simulink model "saved3"  (R2018b)
settings: Solver=VariableStepAuto  StartTime=0.0  StopTime=10.0  RelTol=1e-3
libraries: simulink x95, powerlib x8, powerlib_meascontrol x2
(part 6 of 6)

== matlab function saved3/全观测角速度闭环控制/controller1/MATLAB Function1 ==
  data: u input; y output; t input
function y = fcn(u,t)
startTime=0.2;
if t>startTime
    y=u;
else
    y=0;
end

== matlab function saved3/离散化半成品/PSMS/PMSM dq/MATLAB Function1 ==
  data: i1 input; dw output; i2 input; w input; torE input
function dw = fcn(i1,i2,w,torE)
L1=1e-3; L2=1.4e-3;
phi=0.05;
J=1e-3;
xi=5e-4;

dw = 1/J*(1.5*(phi*i2+(L1-L2)*i1*i2)-xi*w-torE);

== matlab function saved3/全观测角速度闭环控制/w estimater1/MATLAB Function ==
  data: Ea input; y output; Eb input
function y = fcn(Ea,Eb)
if Ea^2+Eb^2<1e-1
    y=0;
else
    y = atan2(Ea,-Eb);
end

== matlab function saved3/全观测角速度闭环控制/w estimater1/clack ==
  data: ia input; iap output; ib input; ic input; ibe output
function [iap,ibe] = fcn(ia,ib,ic)
clack=2/3*[1 -1/2 -1/2;0 sqrt(3)/2 -sqrt(3)/2];
temp=clack*[ia;ib;ic];
iap=temp(1);
ibe=temp(2);

== matlab function saved3/全观测角速度闭环控制/w estimater1/invpark ==
  data: u1 input; ua output; u2 input; ub output; t input
function [ua,ub] = fcn(u1,u2,t)
invPark=[cos(t) -sin(t);sin(t) cos(t)];
temp=invPark*[u1;u2];
ua=temp(1);
ub=temp(2);

== matlab function saved3/离散化半成品/PSMS/clack & park ==
  data: ua input; u1 output; ub input; uc input; t input; u2 output
function [u1,u2] = fcn(ua,ub,uc,t)
clack=2/3*[1 -1/2 -1/2;0 sqrt(3)/2 -sqrt(3)/2];
park=[cos(t) sin(t);-sin(t) cos(t)];
temp=park*clack*[ua;ub;uc];
u1=temp(1);
u2=temp(2);

== matlab function saved3/离散化半成品/PSMS/inv(clack & park) ==
  data: u1 input; ua output; u2 input; t input; ub output; uc output
function [ua,ub,uc] = fcn(u1,u2,t)
invClack=3/2*[2/3 0;-1/3 sqrt(3)/3;-1/3 -sqrt(3)/3];
invPark=[cos(t) -sin(t);sin(t) cos(t)];
temp=invClack*invPark*[u1;u2];
ua=temp(1);
ub=temp(2);
uc=temp(3);

== matlab function saved3/离散化半成品/clack & park2 ==
  data: ua input; u1 output; ub input; uc input; t input; u2 output
function [u1,u2] = fcn(ua,ub,uc,t)
clack=2/3*[1 -1/2 -1/2;0 sqrt(3)/2 -sqrt(3)/2];
park=[cos(t) sin(t);-sin(t) cos(t)];
temp=park*clack*[ua;ub;uc];
u1=temp(1);
u2=temp(2);

== matlab function saved3/离散化半成品/controller/MATLAB Function ==
  data: wloop input; Vdirect input; Switch input; t input; out output
function out = fcn(wloop,Vdirect,Switch,t)
step1time=0.1;
step2time=0.2;
Ustart=1;
direction=1;
if t<step1time
    y=0;
else
    switch Switch
        case 0
            if t<step2time
                y=Ustart*direction;
            else
                y=wloop;
            end
        case 1
            y=Vdirect;
        otherwise
            y=0;
    end
end
out=y;

== matlab function saved3/离散化半成品/controller/MATLAB Function1 ==
  data: u input; y output; t input
function y = fcn(u,t)
startTime=0.2;
if t>startTime
    y=u;
else
    y=0;
end

== matlab function saved3/离散化半成品/inject estimater(digital)/鉴幅鉴相器(可选快速门滑窗) ==
  data: S1 input; A1 output; A2 output; S2 input; DP output; Fre input
function [A1,A2, DP] = fcn(S1,S2,Fre)
Ts=1e-4; %采样时间，其倒数需大于10倍探测信号频率
detPsi=Fre; %探测频率.需采样完整周期整数倍
LowPsi=Fre; %输入信号中的最低显著频率，若探测频率远大于该项，需前置高通滤波器
bufsize=2/LowPsi/Ts;
winSize=1; %滑窗步长
complexStyle=1+1j;
persistent buf1 buf2 round outBuf corebuf gate
if isempty(buf1)||isempty(round)
    buf1=zeros(1,bufsize);
    buf2=zeros(1,bufsize);
    corebuf=zeros(1,bufsize,'like',complexStyle);
    round=0;
    outBuf=[0,0,0];
    gate=0;
end
% 数据读取
if round>=bufsize
    round=0;
    gate=1;
end
buf1(round+1)=S1;
buf2(round+1)=S2;
% 数据处理
corebuf(round+1)=exp(-2*pi*1j*detPsi*round*Ts)*Ts;
if gate==1
    if mod(round+1,winSize)==0
        F1=0+0j;F2=0+0j;
        for n=0:bufsize-1
            F1=F1+buf1(n+1)*corebuf(n+1);
            F2=F2+buf2(n+1)*corebuf(n+1);
        end
        F1=F1*2/bufsize/Ts;F2=F2*2/bufsize/Ts;
        outBuf(1)=norm(F1);outBuf(2)=norm(F2);
        outBuf(3)=angle(F2/F1)*180/pi; %S2超前S1的相位
    end
end
% 更新与输出
round=round+1;
A1=outBuf(1);A2=outBuf(2);
DP=outBuf(3);

== matlab function saved3/离散化半成品/inject estimater(digital)/锁相器 ==
  data: u input; the output; w output
function [the,w] = fcn(u)
% PI控制器部分
ts=1e-4;
kp=4; ki=350;
persistent intg
if isempty(intg)
    intg=0;
end
intg=intg+u*ts;
w = kp*u+ki*intg;

% 积分器部分
persistent intg2
if isempty(intg2)
    intg2=0;
end
intg2=intg2+w*ts;
the = intg2;

== matlab function saved3/离散化半成品/inv(clack & park)1 ==
  data: u1 input; ua output; u2 input; t input; ub output; uc output
function [ua,ub,uc] = fcn(u1,u2,t)
invClack=3/2*[2/3 0;-1/3 sqrt(3)/3;-1/3 -sqrt(3)/3];
invPark=[cos(t) -sin(t);sin(t) cos(t)];
temp=invClack*invPark*[u1;u2];
ua=temp(1);
ub=temp(2);
uc=temp(3);

== matlab function saved3/离散化半成品/w estimater/MATLAB Function ==
  data: Ea input; y output; Eb input
function y = fcn(Ea,Eb)
if Ea^2+Eb^2<1e-1
    y=0;
else
    y = atan2(Ea,-Eb);
end

== matlab function saved3/离散化半成品/w estimater/clack ==
  data: ia input; iap output; ib input; ic input; ibe output
function [iap,ibe] = fcn(ia,ib,ic)
clack=2/3*[1 -1/2 -1/2;0 sqrt(3)/2 -sqrt(3)/2];
temp=clack*[ia;ib;ic];
iap=temp(1);
ibe=temp(2);

== matlab function saved3/离散化半成品/w estimater/invpark ==
  data: u1 input; ua output; u2 input; ub output; t input
function [ua,ub] = fcn(u1,u2,t)
invPark=[cos(t) -sin(t);sin(t) cos(t)];
temp=invPark*[u1;u2];
ua=temp(1);
ub=temp(2);

== matlab function saved3/离散化半成品/电流采样/A//D转换 10KHz2 ==
  data: u input; y output
function y = fcn(u)
bina=16; %二进制位数
deci=2; %小数位数
Max=2^bina;
uper=Max/10^deci/2;
out=fix(u*10^deci+0.5)/10^deci;
y = min(uper,abs(out))*sign(out);

== matlab function saved3/离散化半成品/电流采样/A//D转换 10KHz3 ==
  data: u input; y output
function y = fcn(u)
bina=16; %二进制位数
deci=2; %小数位数
Max=2^bina;
uper=Max/10^deci/2;
out=fix(u*10^deci+0.5)/10^deci;
y = min(uper,abs(out))*sign(out);

== matlab function saved3/离散化半成品/电流采样/A//D转换 10KHz4 ==
  data: u input; y output
function y = fcn(u)
bina=16; %二进制位数
deci=2; %小数位数
Max=2^bina;
uper=Max/10^deci/2;
out=fix(u*10^deci+0.5)/10^deci;
y = min(uper,abs(out))*sign(out);

== matlab function saved3/离散化半成品/电流采样/一阶滤波器40kHz1 ==
  data: u input; y output
function y = fcn(u)
ts=2.5e-5;
N=16000; %截止角频率
persistent xK_1
if isempty(xK_1)
    xK_1=0;
end
x=ts*N*(u-xK_1)+xK_1;
xK_1=x;
y = x;

== matlab function saved3/离散化半成品/电流采样/一阶滤波器40kHz2 ==
  data: u input; y output
function y = fcn(u)
ts=2.5e-5;
N=16000; %截止角频率
persistent xK_1
if isempty(xK_1)
    xK_1=0;
end
x=ts*N*(u-xK_1)+xK_1;
xK_1=x;
y = x;

== matlab function saved3/离散化半成品/电流采样/一阶滤波器40kHz3 ==
  data: u input; y output
function y = fcn(u)
ts=2.5e-5;
N=16000; %截止角频率
persistent xK_1
if isempty(xK_1)
    xK_1=0;
end
x=ts*N*(u-xK_1)+xK_1;
xK_1=x;
y = x;

== matlab function saved3/离散化半成品/2pi 限制2 ==
  data: u input; y output
function y = fcn(u)

y = mod((u+pi),2*pi)-pi;

== matlab function saved3/离散化半成品/MATLAB Function1 ==
  data: hfi input; mlo input; theHat output; t input
function theHat = fcn(hfi, mlo, t)
if t>0.4
    theHat=mlo;
else
    theHat=hfi;
end

== matlab function saved3/离散化半成品/MATLAB Function4 ==
  data: t input; y output
function y = fcn(t)
t=t-0.05;
y = 0*(t<=0.05)+500*(t-0.05)*(0.05<t&&t<=0.35)+(250*(t-0.35)+150)*(0.35<t&&t<=0.55)+200*(t>0.55);

== matlab function saved3/离散化半成品/PSMS1/PMSM dq/MATLAB Function ==
  data: u1 input; di1 output; u2 input; i1 input; i2 input; w input; di2 output
function [di1,di2] = fcn(u1,u2,i1,i2,w)
R=0.1; L1=1e-3; L2=1.4e-3;
phi=0.05;

A=[R/L1 -L2/L1*w;L1/L2*w R/L2];
Y=[1/L1 0;0 1/L2];
I=[i1;i2];
U=[u1;u2];

dI=-A*I+Y*U-phi*w*[0;1/L2];
di1=dI(1);
di2=dI(2);

== matlab function saved3/离散化半成品/PSMS1/PMSM dq/MATLAB Function1 ==
  data: i1 input; dw output; i2 input; w input; torE input
function dw = fcn(i1,i2,w,torE)
L1=1e-3; L2=1.4e-3;
phi=0.05;
J=1e-3;
xi=5e-4;

dw = 1/J*(1.5*(phi*i2+(L1-L2)*i1*i2)-xi*w-torE);

== matlab function saved3/离散化半成品/PSMS1/clack & park ==
  data: ua input; u1 output; ub input; uc input; t input; u2 output
function [u1,u2] = fcn(ua,ub,uc,t)
clack=2/3*[1 -1/2 -1/2;0 sqrt(3)/2 -sqrt(3)/2];
park=[cos(t) sin(t);-sin(t) cos(t)];
temp=park*clack*[ua;ub;uc];
u1=temp(1);
u2=temp(2);

== matlab function saved3/离散化半成品/PSMS1/inv(clack & park) ==
  data: u1 input; ua output; u2 input; t input; ub output; uc output
function [ua,ub,uc] = fcn(u1,u2,t)
invClack=3/2*[2/3 0;-1/3 sqrt(3)/3;-1/3 -sqrt(3)/3];
invPark=[cos(t) -sin(t);sin(t) cos(t)];
temp=invClack*invPark*[u1;u2];
ua=temp(1);
ub=temp(2);
uc=temp(3);

== matlab function saved3/离散化半成品/controller1/MATLAB Function ==
  data: wloop input; Vdirect input; Switch input; t input; out output
function out = fcn(wloop,Vdirect,Switch,t)
step1time=0.1;
step2time=0.2;
Ustart=1;
direction=1;
if t<step1time
    y=0;
else
    switch Switch
        case 0
            if t<step2time
                y=Ustart*direction;
            else
                y=wloop;
            end
        case 1
            y=Vdirect;
        otherwise
            y=0;
    end
end
out=y;

== matlab function saved3/离散化半成品/controller1/MATLAB Function1 ==
  data: u input; y output; t input
function y = fcn(u,t)
startTime=0.2;
if t>startTime
    y=u;
else
    y=0;
end

== matlab function saved3/离散化半成品/controller1/MATLAB Function2 ==
  data: gate input; u input; y output
function y = fcn(gate,u)
if gate<100
    y=u;
else
    y=0;
end

== matlab function saved3/离散化半成品/controller1/clack & park1 ==
  data: ua input; u1 output; ub input; uc input; t input; u2 output
function [u1,u2] = fcn(ua,ub,uc,t)
clack=2/3*[1 -1/2 -1/2;0 sqrt(3)/2 -sqrt(3)/2];
park=[cos(t) sin(t);-sin(t) cos(t)];
temp=park*clack*[ua;ub;uc];
u1=temp(1);
u2=temp(2);

== matlab function saved3/离散化半成品/current seperator/电流采样/A//D转换 10KHz2 ==
  data: u input; y output
function y = fcn(u)
bina=16; %二进制位数
deci=3; %小数位数
Max=2^bina;
uper=Max/10^deci/2;
out=fix(u*10^deci+0.5)/10^deci;
y = min(uper,abs(out))*sign(out);

== matlab function saved3/离散化半成品/current seperator/电流采样/A//D转换 10KHz3 ==
  data: u input; y output
function y = fcn(u)
bina=16; %二进制位数
deci=3; %小数位数
Max=2^bina;
uper=Max/10^deci/2;
out=fix(u*10^deci+0.5)/10^deci;
y = min(uper,abs(out))*sign(out);

== matlab function saved3/离散化半成品/current seperator/电流采样/A//D转换 10KHz4 ==
  data: u input; y output
function y = fcn(u)
bina=16; %二进制位数
deci=3; %小数位数
Max=2^bina;
uper=Max/10^deci/2;
out=fix(u*10^deci+0.5)/10^deci;
y = min(uper,abs(out))*sign(out);

== matlab function saved3/离散化半成品/current seperator/电流采样1/A//D转换 10KHz2 ==
  data: u input; y output
function y = fcn(u)
bina=16; %二进制位数
deci=2; %小数位数
Max=2^bina;
uper=Max/10^deci/2;
out=fix(u*10^deci+0.5)/10^deci;
y = min(uper,abs(out))*sign(out);

== matlab function saved3/离散化半成品/current seperator/电流采样1/A//D转换 10KHz3 ==
  data: u input; y output
function y = fcn(u)
bina=16; %二进制位数
deci=2; %小数位数
Max=2^bina;
uper=Max/10^deci/2;
out=fix(u*10^deci+0.5)/10^deci;
y = min(uper,abs(out))*sign(out);

== matlab function saved3/离散化半成品/current seperator/电流采样1/A//D转换 10KHz4 ==
  data: u input; y output
function y = fcn(u)
bina=16; %二进制位数
deci=2; %小数位数
Max=2^bina;
uper=Max/10^deci/2;
out=fix(u*10^deci+0.5)/10^deci;
y = min(uper,abs(out))*sign(out);

== matlab function saved3/离散化半成品/inject estimater(digital)1/clack & park2 ==
  data: ua input; u1 output; ub input; uc input; t input; u2 output
function [u1,u2] = fcn(ua,ub,uc,t)
clack=2/3*[1 -1/2 -1/2;0 sqrt(3)/2 -sqrt(3)/2];
park=[cos(t) sin(t);-sin(t) cos(t)];
temp=park*clack*[ua;ub;uc];
u1=temp(1);
u2=temp(2);

== matlab function saved3/离散化半成品/inject estimater(digital)1/鉴幅鉴相器(可选快速门滑窗)1 ==
  data: S1 input; A1 output; A2 output; S2 input; DP output; Fre input
function [A1,A2, DP] = fcn(S1,S2,Fre)
Ts=1e-4; %采样时间，其倒数需大于10倍探测信号频率
detPsi=Fre; %探测频率.需采样完整周期整数倍
LowPsi=Fre; %输入信号中的最低显著频率，若探测频率远大于该项，需前置高通滤波器
bufsize=2/LowPsi/Ts;
winSize=1; %滑窗步长
complexStyle=1+1j;
persistent buf1 buf2 round outBuf corebuf gate
if isempty(buf1)||isempty(round)
    buf1=zeros(1,bufsize);
    buf2=zeros(1,bufsize);
    corebuf=zeros(1,bufsize,'like',complexStyle);
    round=0;
    outBuf=[0,0,0];
    gate=0;
end
% 数据读取
if round>=bufsize
    round=0;
    gate=1;
end
buf1(round+1)=S1;
buf2(round+1)=S2;
% 数据处理
corebuf(round+1)=exp(-2*pi*1j*detPsi*round*Ts)*Ts;
if gate==1
    if mod(round+1,winSize)==0
        F1=0+0j;F2=0+0j;
        for n=0:bufsize-1
            F1=F1+buf1(n+1)*corebuf(n+1);
            F2=F2+buf2(n+1)*corebuf(n+1);
        end
        F1=F1*2/bufsize/Ts;F2=F2*2/bufsize/Ts;
        outBuf(1)=norm(F1);outBuf(2)=norm(F2);
        outBuf(3)=angle(F2/F1)*180/pi; %S2超前S1的相位
    end
end
% 更新与输出
round=round+1;
A1=outBuf(1);A2=outBuf(2);
DP=outBuf(3);

== matlab function saved3/离散化半成品/inject estimater(digital)1/锁相器1 ==
  data: u input; the output; w output
function [the,w] = fcn(u)
% PI控制器部分
ts=1e-4;
kp=4; ki=350;
persistent intg
if isempty(intg)
    intg=0;
end
intg=intg+u*ts;
w = kp*u+ki*intg;

% 积分器部分
persistent intg2
if isempty(intg2)
    intg2=0;
end
intg2=intg2+w*ts;
the = intg2;

== matlab function saved3/离散化半成品/inv(clack & park)2 ==
  data: u1 input; ua output; u2 input; t input; ub output; uc output
function [ua,ub,uc] = fcn(u1,u2,t)
invClack=3/2*[2/3 0;-1/3 sqrt(3)/3;-1/3 -sqrt(3)/3];
invPark=[cos(t) -sin(t);sin(t) cos(t)];
temp=invClack*invPark*[u1;u2];
ua=temp(1);
ub=temp(2);
uc=temp(3);

== matlab function saved3/离散化半成品/w estimater1/clack1 ==
  data: ia input; iap output; ib input; ic input; ibe output
function [iap,ibe] = fcn(ia,ib,ic)
clack=2/3*[1 -1/2 -1/2;0 sqrt(3)/2 -sqrt(3)/2];
temp=clack*[ia;ib;ic];
iap=temp(1);
ibe=temp(2);

== matlab function saved3/离散化半成品/2pi 限制3 ==
  data: u input; y output
function y = fcn(u)

y = mod((u+pi),2*pi)-pi;

== matlab function saved3/离散化半成品/MATLAB Function2 ==
  data: t input; y output
function y = fcn(t)
t=t-0.05;
y = 0*(t<=0.05)+500*(t-0.05)*(0.05<t&&t<=0.35)+(250*(t-0.35)+150)*(0.35<t&&t<=0.55)+200*(t>0.55);

== matlab function saved3/离散化半成品/PSMS2/PMSM dq/MATLAB Function ==
  data: u1 input; di1 output; u2 input; i1 input; i2 input; w input; di2 output
function [di1,di2] = fcn(u1,u2,i1,i2,w)
R=0.1; L1=1e-3; L2=1.4e-3;
phi=0.05;

A=[R/L1 -L2/L1*w;L1/L2*w R/L2];
Y=[1/L1 0;0 1/L2];
I=[i1;i2];
U=[u1;u2];

dI=-A*I+Y*U-phi*w*[0;1/L2];
di1=dI(1);
di2=dI(2);

== matlab function saved3/离散化半成品/PSMS2/PMSM dq/MATLAB Function1 ==
  data: i1 input; dw output; i2 input; w input; torE input
function dw = fcn(i1,i2,w,torE)
L1=1e-3; L2=1.4e-3;
phi=0.05;
J=1e-3;
xi=5e-4;

dw = 1/J*(1.5*(phi*i2+(L1-L2)*i1*i2)-xi*w-torE);

== matlab function saved3/离散化半成品/PSMS2/clack & park ==
  data: ua input; u1 output; ub input; uc input; t input; u2 output
function [u1,u2] = fcn(ua,ub,uc,t)
clack=2/3*[1 -1/2 -1/2;0 sqrt(3)/2 -sqrt(3)/2];
park=[cos(t) sin(t);-sin(t) cos(t)];
temp=park*clack*[ua;ub;uc];
u1=temp(1);
u2=temp(2);

== matlab function saved3/离散化半成品/PSMS2/inv(clack & park) ==
  data: u1 input; ua output; u2 input; t input; ub output; uc output
function [ua,ub,uc] = fcn(u1,u2,t)
invClack=3/2*[2/3 0;-1/3 sqrt(3)/3;-1/3 -sqrt(3)/3];
invPark=[cos(t) -sin(t);sin(t) cos(t)];
temp=invClack*invPark*[u1;u2];
ua=temp(1);
ub=temp(2);
uc=temp(3);

== matlab function saved3/离散化半成品/Subsystem/电流采样/A//D转换 10KHz2 ==
  data: u input; y output
function y = fcn(u)
bina=16; %二进制位数
deci=2; %小数位数
Max=2^bina;
uper=Max/10^deci/2;
out=fix(u*10^deci+0.5)/10^deci;
y = min(uper,abs(out))*sign(out);

== matlab function saved3/离散化半成品/Subsystem/电流采样/A//D转换 10KHz3 ==
  data: u input; y output
function y = fcn(u)
bina=16; %二进制位数
deci=2; %小数位数
Max=2^bina;
uper=Max/10^deci/2;
out=fix(u*10^deci+0.5)/10^deci;
y = min(uper,abs(out))*sign(out);

== matlab function saved3/离散化半成品/Subsystem/电流采样/A//D转换 10KHz4 ==
  data: u input; y output
function y = fcn(u)
bina=16; %二进制位数
deci=2; %小数位数
Max=2^bina;
uper=Max/10^deci/2;
out=fix(u*10^deci+0.5)/10^deci;
y = min(uper,abs(out))*sign(out);

== matlab function saved3/离散化半成品/Subsystem/电流采样/一阶滤波器40kHz1 ==
  data: u input; y output
function y = fcn(u)
ts=2.5e-5;
N=16000; %截止角频率
persistent xK_1
if isempty(xK_1)
    xK_1=0;
end
x=ts*N*(u-xK_1)+xK_1;
xK_1=x;
y = x;

== matlab function saved3/离散化半成品/Subsystem/电流采样/一阶滤波器40kHz2 ==
  data: u input; y output
function y = fcn(u)
ts=2.5e-5;
N=16000; %截止角频率
persistent xK_1
if isempty(xK_1)
    xK_1=0;
end
x=ts*N*(u-xK_1)+xK_1;
xK_1=x;
y = x;

== matlab function saved3/离散化半成品/Subsystem/电流采样/一阶滤波器40kHz3 ==
  data: u input; y output
function y = fcn(u)
ts=2.5e-5;
N=16000; %截止角频率
persistent xK_1
if isempty(xK_1)
    xK_1=0;
end
x=ts*N*(u-xK_1)+xK_1;
xK_1=x;
y = x;

== matlab function saved3/离散化半成品/clack & park1 ==
  data: ua input; u1 output; ub input; uc input; t input; u2 output
function [u1,u2] = fcn(ua,ub,uc,t)
clack=2/3*[1 -1/2 -1/2;0 sqrt(3)/2 -sqrt(3)/2];
park=[cos(t) sin(t);-sin(t) cos(t)];
temp=park*clack*[ua;ub;uc];
u1=temp(1);
u2=temp(2);

== matlab function saved3/离散化半成品/controller2/MATLAB Function ==
  data: wloop input; Vdirect input; Switch input; t input; out output
function out = fcn(wloop,Vdirect,Switch,t)
step1time=0.1;
step2time=0.2;
Ustart=1;
direction=1;
if t<step1time
    y=0;
else
    switch Switch
        case 0
            if t<step2time
                y=Ustart*direction;
            else
                y=wloop;
            end
        case 1
            y=Vdirect;
        otherwise
            y=0;
    end
end
out=y;

== matlab function saved3/离散化半成品/controller2/MATLAB Function1 ==
  data: u input; y output; t input
function y = fcn(u,t)
startTime=0.2;
if t>startTime
    y=u;
else
    y=0;
end

== matlab function saved3/离散化半成品/inject estimater(digital)2/clack & park2 ==
  data: ua input; u1 output; ub input; uc input; t input; u2 output
function [u1,u2] = fcn(ua,ub,uc,t)
clack=2/3*[1 -1/2 -1/2;0 sqrt(3)/2 -sqrt(3)/2];
park=[cos(t) sin(t);-sin(t) cos(t)];
temp=park*clack*[ua;ub;uc];
u1=temp(1);
u2=temp(2);

== matlab function saved3/离散化半成品/inject estimater(digital)2/鉴幅鉴相器(可选快速门滑窗)1 ==
  data: S1 input; A1 output; A2 output; S2 input; DP output; Fre input
function [A1,A2, DP] = fcn(S1,S2,Fre)
Ts=1e-4; %采样时间，其倒数需大于10倍探测信号频率
detPsi=Fre; %探测频率.需采样完整周期整数倍
LowPsi=Fre; %输入信号中的最低显著频率，若探测频率远大于该项，需前置高通滤波器
bufsize=2/LowPsi/Ts;
winSize=1; %滑窗步长
complexStyle=1+1j;
persistent buf1 buf2 round outBuf corebuf gate
if isempty(buf1)||isempty(round)
    buf1=zeros(1,bufsize);
    buf2=zeros(1,bufsize);
    corebuf=zeros(1,bufsize,'like',complexStyle);
    round=0;
    outBuf=[0,0,0];
    gate=0;
end
% 数据读取
if round>=bufsize
    round=0;
    gate=1;
end
buf1(round+1)=S1;
buf2(round+1)=S2;
% 数据处理
corebuf(round+1)=exp(-2*pi*1j*detPsi*round*Ts)*Ts;
if gate==1
    if mod(round+1,winSize)==0
        F1=0+0j;F2=0+0j;
        for n=0:bufsize-1
            F1=F1+buf1(n+1)*corebuf(n+1);
            F2=F2+buf2(n+1)*corebuf(n+1);
        end
        F1=F1*2/bufsize/Ts;F2=F2*2/bufsize/Ts;
        outBuf(1)=norm(F1);outBuf(2)=norm(F2);
        outBuf(3)=angle(F2/F1)*180/pi; %S2超前S1的相位
    end
end
% 更新与输出
round=round+1;
A1=outBuf(1);A2=outBuf(2);
DP=outBuf(3);

== matlab function saved3/离散化半成品/inject estimater(digital)2/锁相器1 ==
  data: u input; the output; w output
function [the,w] = fcn(u)
% PI控制器部分
ts=1e-4;
kp=4; ki=350;
persistent intg
if isempty(intg)
    intg=0;
end
intg=intg+u*ts;
w = kp*u+ki*intg;

% 积分器部分
persistent intg2
if isempty(intg2)
    intg2=0;
end
intg2=intg2+w*ts;
the = intg2;

== matlab function saved3/离散化半成品/inv(clack & park)3 ==
  data: u1 input; ua output; u2 input; t input; ub output; uc output
function [ua,ub,uc] = fcn(u1,u2,t)
invClack=3/2*[2/3 0;-1/3 sqrt(3)/3;-1/3 -sqrt(3)/3];
invPark=[cos(t) -sin(t);sin(t) cos(t)];
temp=invClack*invPark*[u1;u2];
ua=temp(1);
ub=temp(2);
uc=temp(3);

== matlab function saved3/离散化半成品/w estimater2/MATLAB Function ==
  data: Ea input; y output; Eb input
function y = fcn(Ea,Eb)
if Ea^2+Eb^2<1e-1
    y=0;
else
    y = atan2(Ea,-Eb);
end

== matlab function saved3/离散化半成品/w estimater2/clack ==
  data: ia input; iap output; ib input; ic input; ibe output
function [iap,ibe] = fcn(ia,ib,ic)
clack=2/3*[1 -1/2 -1/2;0 sqrt(3)/2 -sqrt(3)/2];
temp=clack*[ia;ib;ic];
iap=temp(1);
ibe=temp(2);

== matlab function saved3/离散化半成品/w estimater2/invpark ==
  data: u1 input; ua output; u2 input; ub output; t input
function [ua,ub] = fcn(u1,u2,t)
invPark=[cos(t) -sin(t);sin(t) cos(t)];
temp=invPark*[u1;u2];
ua=temp(1);
ub=temp(2);

== matlab function saved3/离散化半成品/电流采样1/A//D转换 10KHz2 ==
  data: u input; y output
function y = fcn(u)
bina=16; %二进制位数
deci=2; %小数位数
Max=2^bina;
uper=Max/10^deci/2;
out=fix(u*10^deci+0.5)/10^deci;
y = min(uper,abs(out))*sign(out);

== matlab function saved3/离散化半成品/电流采样1/A//D转换 10KHz3 ==
  data: u input; y output
function y = fcn(u)
bina=16; %二进制位数
deci=2; %小数位数
Max=2^bina;
uper=Max/10^deci/2;
out=fix(u*10^deci+0.5)/10^deci;
y = min(uper,abs(out))*sign(out);

== matlab function saved3/离散化半成品/电流采样1/A//D转换 10KHz4 ==
  data: u input; y output
function y = fcn(u)
bina=16; %二进制位数
deci=2; %小数位数
Max=2^bina;
uper=Max/10^deci/2;
out=fix(u*10^deci+0.5)/10^deci;
y = min(uper,abs(out))*sign(out);

== matlab function saved3/离散化半成品/电流采样1/一阶滤波器40kHz1 ==
  data: u input; y output
function y = fcn(u)
ts=2.5e-5;
N=16000; %截止角频率
persistent xK_1
if isempty(xK_1)
    xK_1=0;
end
x=ts*N*(u-xK_1)+xK_1;
xK_1=x;
y = x;

== matlab function saved3/全观测角速度闭环控制/controller/MATLAB Function1 ==
  data: u input; y output; t input
function y = fcn(u,t)
startTime=0.2;
if t>startTime
    y=u;
else
    y=0;
end

== matlab function saved3/离散化半成品/电流采样1/一阶滤波器40kHz2 ==
  data: u input; y output
function y = fcn(u)
ts=2.5e-5;
N=16000; %截止角频率
persistent xK_1
if isempty(xK_1)
    xK_1=0;
end
x=ts*N*(u-xK_1)+xK_1;
xK_1=x;
y = x;

== matlab function saved3/离散化半成品/电流采样1/一阶滤波器40kHz3 ==
  data: u input; y output
function y = fcn(u)
ts=2.5e-5;
N=16000; %截止角频率
persistent xK_1
if isempty(xK_1)
    xK_1=0;
end
x=ts*N*(u-xK_1)+xK_1;
xK_1=x;
y = x;

== matlab function saved3/离散化半成品/MATLAB Function ==
  data: Inj input; theHat output; Emf input; wHat input; t input
function theHat = fcn(Inj,Emf, wHat,t)

if t>0.4
    theHat=Emf;
else
    theHat=Inj;
end

== matlab function saved3/离散化半成品/MATLAB Function3 ==
  data: t input; y output
function y = fcn(t)
t=t-0.05;
y = 0*(t<=0.05)+500*(t-0.05)*(0.05<t&&t<=0.35)+(250*(t-0.35)+150)*(0.35<t&&t<=0.55)+200*(t>0.55);

== matlab function saved3/全观测角速度闭环控制/PSMS/PMSM dq/MATLAB Function ==
  data: u1 input; di1 output; u2 input; i1 input; i2 input; w input; di2 output
function [di1,di2] = fcn(u1,u2,i1,i2,w)
R=0.1; L1=1e-3; L2=1.4e-3;
phi=0.05;

A=[R/L1 -L2/L1*w;L1/L2*w R/L2];
Y=[1/L1 0;0 1/L2];
I=[i1;i2];
U=[u1;u2];

dI=-A*I+Y*U-phi*w*[0;1/L2];
di1=dI(1);
di2=dI(2);

== matlab function saved3/全观测角速度闭环控制/PSMS/PMSM dq/MATLAB Function1 ==
  data: i1 input; dw output; i2 input; w input; torE input
function dw = fcn(i1,i2,w,torE)
L1=1e-3; L2=1.4e-3;
phi=0.05;
J=1e-3;
xi=5e-4;

dw = 1/J*(1.5*(phi*i2+(L1-L2)*i1*i2)-xi*w-torE);

== matlab function saved3/全观测角速度闭环控制/PSMS/clack & park ==
  data: ua input; u1 output; ub input; uc input; t input; u2 output
function [u1,u2] = fcn(ua,ub,uc,t)
clack=2/3*[1 -1/2 -1/2;0 sqrt(3)/2 -sqrt(3)/2];
park=[cos(t) sin(t);-sin(t) cos(t)];
temp=park*clack*[ua;ub;uc];
u1=temp(1);
u2=temp(2);

== matlab function saved3/全观测角速度闭环控制/PSMS/inv(clack & park) ==
  data: u1 input; ua output; u2 input; t input; ub output; uc output
function [ua,ub,uc] = fcn(u1,u2,t)
invClack=3/2*[2/3 0;-1/3 sqrt(3)/3;-1/3 -sqrt(3)/3];
invPark=[cos(t) -sin(t);sin(t) cos(t)];
temp=invClack*invPark*[u1;u2];
ua=temp(1);
ub=temp(2);
uc=temp(3);

== matlab function saved3/全观测角速度闭环控制/clack & park2 ==
  data: ua input; u1 output; ub input; uc input; t input; u2 output
function [u1,u2] = fcn(ua,ub,uc,t)
clack=2/3*[1 -1/2 -1/2;0 sqrt(3)/2 -sqrt(3)/2];
park=[cos(t) sin(t);-sin(t) cos(t)];
temp=park*clack*[ua;ub;uc];
u1=temp(1);
u2=temp(2);

== matlab function saved3/离散化半成品/PSMS3/PMSM dq/MATLAB Function ==
  data: u1 input; di1 output; u2 input; i1 input; i2 input; w input; di2 output
function [di1,di2] = fcn(u1,u2,i1,i2,w)
R=0.1; L1=1e-3; L2=1.4e-3;
phi=0.05;

A=[R/L1 -L2/L1*w;L1/L2*w R/L2];
Y=[1/L1 0;0 1/L2];
I=[i1;i2];
U=[u1;u2];

dI=-A*I+Y*U-phi*w*[0;1/L2];
di1=dI(1);
di2=dI(2);

== matlab function saved3/全观测角速度闭环控制/inv(clack & park)1 ==
  data: u1 input; ua output; u2 input; t input; ub output; uc output
function [ua,ub,uc] = fcn(u1,u2,t)
invClack=3/2*[2/3 0;-1/3 sqrt(3)/3;-1/3 -sqrt(3)/3];
invPark=[cos(t) -sin(t);sin(t) cos(t)];
temp=invClack*invPark*[u1;u2];
ua=temp(1);
ub=temp(2);
uc=temp(3);

== matlab function saved3/离散化半成品/PSMS3/PMSM dq/MATLAB Function1 ==
  data: i1 input; dw output; i2 input; w input; torE input
function dw = fcn(i1,i2,w,torE)
L1=1e-3; L2=1.4e-3;
phi=0.05;
J=1e-3;
xi=5e-4;

dw = 1/J*(1.5*(phi*i2+(L1-L2)*i1*i2)-xi*w-torE);

== matlab function saved3/离散化半成品/PSMS3/clack & park ==
  data: ua input; u1 output; ub input; uc input; t input; u2 output
function [u1,u2] = fcn(ua,ub,uc,t)
clack=2/3*[1 -1/2 -1/2;0 sqrt(3)/2 -sqrt(3)/2];
park=[cos(t) sin(t);-sin(t) cos(t)];
temp=park*clack*[ua;ub;uc];
u1=temp(1);
u2=temp(2);

== matlab function saved3/离散化半成品/PSMS3/inv(clack & park) ==
  data: u1 input; ua output; u2 input; t input; ub output; uc output
function [ua,ub,uc] = fcn(u1,u2,t)
invClack=3/2*[2/3 0;-1/3 sqrt(3)/3;-1/3 -sqrt(3)/3];
invPark=[cos(t) -sin(t);sin(t) cos(t)];
temp=invClack*invPark*[u1;u2];
ua=temp(1);
ub=temp(2);
uc=temp(3);

== matlab function saved3/离散化半成品/Subsystem1/2pi 限制1 ==
  data: u input; y output
function y = fcn(u)

y = mod((u+pi),2*pi)-pi;

== matlab function saved3/离散化半成品/Subsystem1/2pi 限制2 ==
  data: u input; y output
function y = fcn(u)

y = mod((u+pi),2*pi)-pi;

== matlab function saved3/离散化半成品/clack & park3 ==
  data: ua input; u1 output; ub input; uc input; t input; u2 output
function [u1,u2] = fcn(ua,ub,uc,t)
clack=2/3*[1 -1/2 -1/2;0 sqrt(3)/2 -sqrt(3)/2];
park=[cos(t) sin(t);-sin(t) cos(t)];
temp=park*clack*[ua;ub;uc];
u1=temp(1);
u2=temp(2);

== matlab function saved3/离散化半成品/controller3/MATLAB Function ==
  data: wloop input; Vdirect input; Switch input; t input; out output
function out = fcn(wloop,Vdirect,Switch,t)
step1time=0.1;
step2time=0.2;
Ustart=1;
direction=1;
if t<step1time
    y=0;
else
    switch Switch
        case 0
            if t<step2time
                y=Ustart*direction;
            else
                y=wloop;
            end
        case 1
            y=Vdirect;
        otherwise
            y=0;
    end
end
out=y;

== matlab function saved3/离散化半成品/controller3/MATLAB Function1 ==
  data: u input; y output; t input
function y = fcn(u,t)
startTime=0.2;
if t>startTime
    y=u;
else
    y=0;
end

== matlab function saved3/离散化半成品/inject estimater(digital)3/鉴幅鉴相器(可选快速门滑窗) ==
  data: S1 input; A1 output; A2 output; S2 input; DP output; Fre input
function [A1,A2, DP] = fcn(S1,S2,Fre)
Ts=1e-4; %采样时间，其倒数需大于10倍探测信号频率
detPsi=Fre; %探测频率.需采样完整周期整数倍
LowPsi=Fre; %输入信号中的最低显著频率，若探测频率远大于该项，需前置高通滤波器
bufsize=2/LowPsi/Ts;
winSize=1; %滑窗步长
complexStyle=1+1j;
persistent buf1 buf2 round outBuf corebuf gate
if isempty(buf1)||isempty(round)
    buf1=zeros(1,bufsize);
    buf2=zeros(1,bufsize);
    corebuf=zeros(1,bufsize,'like',complexStyle);
    round=0;
    outBuf=[0,0,0];
    gate=0;
end
% 数据读取
if round>=bufsize
    round=0;
    gate=1;
end
buf1(round+1)=S1;
buf2(round+1)=S2;
% 数据处理
corebuf(round+1)=exp(-2*pi*1j*detPsi*round*Ts)*Ts;
if gate==1
    if mod(round+1,winSize)==0
        F1=0+0j;F2=0+0j;
        for n=0:bufsize-1
            F1=F1+buf1(n+1)*corebuf(n+1);
            F2=F2+buf2(n+1)*corebuf(n+1);
        end
        F1=F1*2/bufsize/Ts;F2=F2*2/bufsize/Ts;
        outBuf(1)=norm(F1);outBuf(2)=norm(F2);
        outBuf(3)=angle(F2/F1)*180/pi; %S2超前S1的相位
    end
end
% 更新与输出
round=round+1;
A1=outBuf(1);A2=outBuf(2);
DP=outBuf(3);

== matlab function saved3/离散化半成品/inject estimater(digital)3/锁相器 ==
  data: u input; the output; w output
function [the,w] = fcn(u)
% PI控制器部分
ts=1e-4;
kp=4; ki=350;
persistent intg
if isempty(intg)
    intg=0;
end
intg=intg+u*ts;
w = kp*u+ki*intg;

% 积分器部分
persistent intg2
if isempty(intg2)
    intg2=0;
end
intg2=intg2+w*ts;
the = intg2;

== matlab function saved3/离散化半成品/inv(clack & park)4 ==
  data: u1 input; ua output; u2 input; t input; ub output; uc output
function [ua,ub,uc] = fcn(u1,u2,t)
invClack=3/2*[2/3 0;-1/3 sqrt(3)/3;-1/3 -sqrt(3)/3];
invPark=[cos(t) -sin(t);sin(t) cos(t)];
temp=invClack*invPark*[u1;u2];
ua=temp(1);
ub=temp(2);
uc=temp(3);

== matlab function saved3/离散化半成品/w estimater3/MATLAB Function ==
  data: Ea input; y output; Eb input
function y = fcn(Ea,Eb)
if Ea^2+Eb^2<1e-1
    y=0;
else
    y = atan2(Ea,-Eb);
end

== matlab function saved3/离散化半成品/w estimater3/clack ==
  data: ia input; iap output; ib input; ic input; ibe output
function [iap,ibe] = fcn(ia,ib,ic)
clack=2/3*[1 -1/2 -1/2;0 sqrt(3)/2 -sqrt(3)/2];
temp=clack*[ia;ib;ic];
iap=temp(1);
ibe=temp(2);

== matlab function saved3/离散化半成品/w estimater3/invpark ==
  data: u1 input; ua output; u2 input; ub output; t input
function [ua,ub] = fcn(u1,u2,t)
invPark=[cos(t) -sin(t);sin(t) cos(t)];
temp=invPark*[u1;u2];
ua=temp(1);
ub=temp(2);

== matlab function saved3/离散化半成品/w estimater3/磁链观测器 ==
  data: u input; y output
function y = fcn(u)
ts=1e-4;
R=0.1;
L=1.2e-3;
Psi_mm=0.1;
uob=[u(1);u(2)];
iob=[u(3);u(4)];

persistent x_1
if isempty(x_1)
    x_1=[0;0];
end
gamma=20000;
ita=x_1-L*iob;
err=Psi_mm^2-norm(ita)^2;
x=x_1 + (uob-iob*R+gamma*ita*err)*ts;
x_1=x;
v=(x-L*iob);
y = atan2(v(2),v(1));

== matlab function saved3/离散化半成品/电流采样2/A//D转换 10KHz2 ==
  data: u input; y output
function y = fcn(u)
bina=16; %二进制位数
deci=2; %小数位数
Max=2^bina;
uper=Max/10^deci/2;
out=fix(u*10^deci+0.5)/10^deci;
y = min(uper,abs(out))*sign(out);

== matlab function saved3/离散化半成品/电流采样2/A//D转换 10KHz3 ==
  data: u input; y output
function y = fcn(u)
bina=16; %二进制位数
deci=2; %小数位数
Max=2^bina;
uper=Max/10^deci/2;
out=fix(u*10^deci+0.5)/10^deci;
y = min(uper,abs(out))*sign(out);

== matlab function saved3/离散化半成品/电流采样2/A//D转换 10KHz4 ==
  data: u input; y output
function y = fcn(u)
bina=16; %二进制位数
deci=2; %小数位数
Max=2^bina;
uper=Max/10^deci/2;
out=fix(u*10^deci+0.5)/10^deci;
y = min(uper,abs(out))*sign(out);

== matlab function saved3/离散化半成品/电流采样2/一阶滤波器40kHz1 ==
  data: u input; y output
function y = fcn(u)
ts=2.5e-5;
N=16000; %截止角频率
persistent xK_1
if isempty(xK_1)
    xK_1=0;
end
x=ts*N*(u-xK_1)+xK_1;
xK_1=x;
y = x;

== matlab function saved3/离散化半成品/电流采样2/一阶滤波器40kHz2 ==
  data: u input; y output
function y = fcn(u)
ts=2.5e-5;
N=16000; %截止角频率
persistent xK_1
if isempty(xK_1)
    xK_1=0;
end
x=ts*N*(u-xK_1)+xK_1;
xK_1=x;
y = x;

== matlab function saved3/全观测角速度闭环控制/MATLAB Function3 ==
  data: ud input; ua output; uq input; t input; ub output
function [ua,ub] = fcn(ud,uq,t)
R=[cos(t) -sin(t);sin(t) cos(t)];
temp=R*[ud;uq];
ua=temp(1);
ub=temp(2);

== matlab function saved3/离散化半成品/电流采样2/一阶滤波器40kHz3 ==
  data: u input; y output
function y = fcn(u)
ts=2.5e-5;
N=16000; %截止角频率
persistent xK_1
if isempty(xK_1)
    xK_1=0;
end
x=ts*N*(u-xK_1)+xK_1;
xK_1=x;
y = x;

== matlab function saved3/离散化半成品/w estimater1/invpark ==
  data: u1 input; ua output; u2 input; ub output; t input
function [ua,ub] = fcn(u1,u2,t)
invPark=[cos(t) -sin(t);sin(t) cos(t)];
temp=invPark*[u1;u2];
ua=temp(1);
ub=temp(2);

== matlab function saved3/离散化半成品/w estimater1/磁链观测器 ==
  data: u input; y output
function y = fcn(u)
ts=1e-4;
R=0.1;
L=1.2e-3;
Psi_mm=0.1;
uob=[u(1);u(2)];
iob=[u(3);u(4)];

persistent x_1
if isempty(x_1)
    x_1=[0;0];
end
gamma=20000;
ita=x_1-L*iob;
err=Psi_mm^2-norm(ita)^2;
x=x_1 + (uob-iob*R+gamma*ita*err)*ts;
x_1=x;
v=(x-L*iob);
y = atan2(v(2),v(1))-0.0;

== matlab function saved3/全观测角速度闭环控制/MATLAB Function7 ==
  data: t input; y output
function y = fcn(t)
t=t-0.05;
y = 0*(t<=0.05)+500*(t-0.05)*(0.05<t&&t<=0.35)+(250*(t-0.35)+150)*(0.35<t&&t<=0.55)+200*(t>0.55);

== matlab function saved3/电压控制离散化/2pi 限制3 ==
  data: u input; y output
function y = fcn(u)

y = mod((u+pi),2*pi)-pi;

== matlab function saved3/电压控制离散化/MATLAB Function ==
  data: hfi input; mlo input; theHat output; t input
function theHat = fcn(hfi, mlo, t)
if t>0.4
    theHat=mlo;
else
    theHat=hfi;
end

== matlab function saved3/电压控制离散化/MATLAB Function2 ==
  data: t input; y output
function y = fcn(t)
t=t-0.05;
y = 0*(t<=0.05)+500*(t-0.05)*(0.05<t&&t<=0.35)+(250*(t-0.35)+150)*(0.35<t&&t<=0.55)+200*(t>0.55);

== matlab function saved3/电压控制离散化/MATLAB Function3 ==
  data: ud input; ua output; uq input; t input; ub output
function [ua,ub] = fcn(ud,uq,t)
R=[cos(t) -sin(t);sin(t) cos(t)];
temp=R*[ud;uq];
ua=temp(1);
ub=temp(2);

== matlab function saved3/全观测角速度闭环控制/clack & park3 ==
  data: ua input; u1 output; ub input; uc input; t input; u2 output
function [u1,u2] = fcn(ua,ub,uc,t)
clack=2/3*[1 -1/2 -1/2;0 sqrt(3)/2 -sqrt(3)/2];
park=[cos(t) sin(t);-sin(t) cos(t)];
temp=park*clack*[ua;ub;uc];
u1=temp(1);
u2=temp(2);

== matlab function saved3/电压控制离散化/controller2/MATLAB Function ==
  data: wloop input; Vdirect input; Switch input; t input; out output
function out = fcn(wloop,Vdirect,Switch,t)
step1time=0.1;
step2time=0.2;
Ustart=1;
direction=1;
if t<step1time
    y=0;
else
    switch Switch
        case 0
            if t<step2time
                y=Ustart*direction;
            else
                y=wloop;
            end
        case 1
            y=Vdirect;
        otherwise
            y=0;
    end
end
out=y;

== matlab function saved3/电压控制离散化/controller2/MATLAB Function1 ==
  data: u input; y output; t input
function y = fcn(u,t)
startTime=0.2;
if t>startTime
    y=u;
else
    y=0;
end

== matlab function saved3/电压控制离散化/controller2/MATLAB Function2 ==
  data: gate input; u input; y output
function y = fcn(gate,u)
if gate<100
    y=u;
else
    y=0;
end

== matlab function saved3/电压控制离散化/controller2/clack & park1 ==
  data: ua input; u1 output; ub input; uc input; t input; u2 output
function [u1,u2] = fcn(ua,ub,uc,t)
clack=2/3*[1 -1/2 -1/2;0 sqrt(3)/2 -sqrt(3)/2];
park=[cos(t) sin(t);-sin(t) cos(t)];
temp=park*clack*[ua;ub;uc];
u1=temp(1);
u2=temp(2);

== matlab function saved3/电压控制离散化/current seperator/电流采样/A//D转换 10KHz2 ==
  data: u input; y output
function y = fcn(u)
bina=16; %二进制位数
deci=3; %小数位数
Max=2^bina;
uper=Max/10^deci/2;
out=fix(u*10^deci+0.5)/10^deci;
y = min(uper,abs(out))*sign(out);

== matlab function saved3/电压控制离散化/current seperator/电流采样/A//D转换 10KHz3 ==
  data: u input; y output
function y = fcn(u)
bina=16; %二进制位数
deci=3; %小数位数
Max=2^bina;
uper=Max/10^deci/2;
out=fix(u*10^deci+0.5)/10^deci;
y = min(uper,abs(out))*sign(out);

== matlab function saved3/全观测角速度闭环控制/电压圆限制 ==
  data: Ua input; ua output; Ub input; ub output
function [ua,ub] = fcn(Ua,Ub)
umax=24/(sqrt(3)/2);
ua=Ua/umax;
ub=Ub/umax;

== matlab function saved3/电压控制离散化/current seperator/电流采样/A//D转换 10KHz4 ==
  data: u input; y output
function y = fcn(u)
bina=16; %二进制位数
deci=3; %小数位数
Max=2^bina;
uper=Max/10^deci/2;
out=fix(u*10^deci+0.5)/10^deci;
y = min(uper,abs(out))*sign(out);

== matlab function saved3/电压控制离散化/current seperator/电流采样1/A//D转换 10KHz2 ==
  data: u input; y output
function y = fcn(u)
bina=16; %二进制位数
deci=2; %小数位数
Max=2^bina;
uper=Max/10^deci/2;
out=fix(u*10^deci+0.5)/10^deci;
y = min(uper,abs(out))*sign(out);

== matlab function saved3/电压控制离散化/current seperator/电流采样1/A//D转换 10KHz3 ==
  data: u input; y output
function y = fcn(u)
bina=16; %二进制位数
deci=2; %小数位数
Max=2^bina;
uper=Max/10^deci/2;
out=fix(u*10^deci+0.5)/10^deci;
y = min(uper,abs(out))*sign(out);

== matlab function saved3/电压控制离散化/current seperator/电流采样1/A//D转换 10KHz4 ==
  data: u input; y output
function y = fcn(u)
bina=16; %二进制位数
deci=2; %小数位数
Max=2^bina;
uper=Max/10^deci/2;
out=fix(u*10^deci+0.5)/10^deci;
y = min(uper,abs(out))*sign(out);

== matlab function saved3/电压控制离散化/inject estimater(digital)2/clack & park2 ==
  data: ua input; u1 output; ub input; uc input; t input; u2 output
function [u1,u2] = fcn(ua,ub,uc,t)
clack=2/3*[1 -1/2 -1/2;0 sqrt(3)/2 -sqrt(3)/2];
park=[cos(t) sin(t);-sin(t) cos(t)];
temp=park*clack*[ua;ub;uc];
u1=temp(1);
u2=temp(2);

== matlab function saved3/电压控制离散化/inject estimater(digital)2/鉴幅鉴相器(可选快速门滑窗)1 ==
  data: S1 input; A1 output; A2 output; S2 input; DP output; Fre input
function [A1,A2, DP] = fcn(S1,S2,Fre)
Ts=1e-4; %采样时间，其倒数需大于10倍探测信号频率
detPsi=Fre; %探测频率.需采样完整周期整数倍
LowPsi=Fre; %输入信号中的最低显著频率，若探测频率远大于该项，需前置高通滤波器
bufsize=2/LowPsi/Ts;
winSize=1; %滑窗步长
complexStyle=1+1j;
persistent buf1 buf2 round outBuf corebuf gate
if isempty(buf1)||isempty(round)
    buf1=zeros(1,bufsize);
    buf2=zeros(1,bufsize);
    corebuf=zeros(1,bufsize,'like',complexStyle);
    round=0;
    outBuf=[0,0,0];
    gate=0;
end
% 数据读取
if round>=bufsize
    round=0;
    gate=1;
end
buf1(round+1)=S1;
buf2(round+1)=S2;
% 数据处理
corebuf(round+1)=exp(-2*pi*1j*detPsi*round*Ts)*Ts;
if gate==1
    if mod(round+1,winSize)==0
        F1=0+0j;F2=0+0j;
        for n=0:bufsize-1
            F1=F1+buf1(n+1)*corebuf(n+1);
            F2=F2+buf2(n+1)*corebuf(n+1);
        end
        F1=F1*2/bufsize/Ts;F2=F2*2/bufsize/Ts;
        outBuf(1)=norm(F1);outBuf(2)=norm(F2);
        outBuf(3)=angle(F2/F1)*180/pi; %S2超前S1的相位
    end
end
% 更新与输出
round=round+1;
A1=outBuf(1);A2=outBuf(2);
DP=outBuf(3);

== matlab function saved3/电压控制离散化/inject estimater(digital)2/锁相器1 ==
  data: u input; the output; w output
function [the,w] = fcn(u)
% PI控制器部分
ts=1e-4;
kp=4; ki=350;
persistent intg
if isempty(intg)
    intg=0;
end
intg=intg+u*ts;
w = kp*u+ki*intg;

% 积分器部分
persistent intg2
if isempty(intg2)
    intg2=0;
end
intg2=intg2+w*ts;
the = intg2;

== matlab function saved3/电压控制离散化/w estimater2/clack1 ==
  data: ia input; iap output; ib input; ic input; ibe output
function [iap,ibe] = fcn(ia,ib,ic)
clack=2/3*[1 -1/2 -1/2;0 sqrt(3)/2 -sqrt(3)/2];
temp=clack*[ia;ib;ic];
iap=temp(1);
ibe=temp(2);

== matlab function saved3/电压控制离散化/w estimater2/invpark ==
  data: u1 input; ua output; u2 input; ub output; t input
function [ua,ub] = fcn(u1,u2,t)
invPark=[cos(t) -sin(t);sin(t) cos(t)];
temp=invPark*[u1;u2];
ua=temp(1);
ub=temp(2);

== matlab function saved3/电压控制离散化/w estimater2/磁链观测器 ==
  data: u input; y output
function y = fcn(u)
ts=1e-4;
R=0.1;
L=1.2e-3;
Psi_mm=0.1;
uob=[u(1);u(2)];
iob=[u(3);u(4)];

persistent x_1
if isempty(x_1)
    x_1=[0;0];
end
gamma=20000;
ita=x_1-L*iob;
err=Psi_mm^2-norm(ita)^2;
x=x_1 + (uob-iob*R+gamma*ita*err)*ts;
x_1=x;
v=(x-L*iob);
y = atan2(v(2),v(1))-0.0;

== matlab function saved3/电压控制离散化/电压圆限制 ==
  data: Ua input; ua output; Ub input; ub output
function [ua,ub] = fcn(Ua,Ub)
umax=24/(sqrt(3)/2);
ua=Ua/umax;
ub=Ub/umax;

== matlab function saved3/电压控制离散化/2pi 限制2 ==
  data: u input; y output
function y = fcn(u)

y = mod((u+pi),2*pi)-pi;

== matlab function saved3/电压控制离散化/MATLAB Function1 ==
  data: hfi input; mlo input; theHat output; t input
function theHat = fcn(hfi, mlo, t)
if t>0.4
    theHat=mlo;
else
    theHat=hfi;
end

== matlab function saved3/电压控制离散化/MATLAB Function4 ==
  data: t input; y output
function y = fcn(t)
t=t-0.05;
y = 0*(t<=0.05)+500*(t-0.05)*(0.05<t&&t<=0.35)+(250*(t-0.35)+150)*(0.35<t&&t<=0.55)+200*(t>0.55);

== matlab function saved3/电压控制离散化/PSMS1/PMSM dq/MATLAB Function ==
  data: u1 input; di1 output; u2 input; i1 input; i2 input; w input; di2 output
function [di1,di2] = fcn(u1,u2,i1,i2,w)
R=0.1; L1=1e-3; L2=1.4e-3;
phi=0.05;

A=[R/L1 -L2/L1*w;L1/L2*w R/L2];
Y=[1/L1 0;0 1/L2];
I=[i1;i2];
U=[u1;u2];

dI=-A*I+Y*U-phi*w*[0;1/L2];
di1=dI(1);
di2=dI(2);

== matlab function saved3/电压控制离散化/PSMS1/PMSM dq/MATLAB Function1 ==
  data: i1 input; dw output; i2 input; w input; torE input
function dw = fcn(i1,i2,w,torE)
L1=1e-3; L2=1.4e-3;
phi=0.05;
J=1e-3;
xi=5e-4;

dw = 1/J*(1.5*(phi*i2+(L1-L2)*i1*i2)-xi*w-torE);

== matlab function saved3/电压控制离散化/PSMS1/clack & park ==
  data: ua input; u1 output; ub input; uc input; t input; u2 output
function [u1,u2] = fcn(ua,ub,uc,t)
clack=2/3*[1 -1/2 -1/2;0 sqrt(3)/2 -sqrt(3)/2];
park=[cos(t) sin(t);-sin(t) cos(t)];
temp=park*clack*[ua;ub;uc];
u1=temp(1);
u2=temp(2);

== matlab function saved3/电压控制离散化/PSMS1/inv(clack & park) ==
  data: u1 input; ua output; u2 input; t input; ub output; uc output
function [ua,ub,uc] = fcn(u1,u2,t)
invClack=3/2*[2/3 0;-1/3 sqrt(3)/3;-1/3 -sqrt(3)/3];
invPark=[cos(t) -sin(t);sin(t) cos(t)];
temp=invClack*invPark*[u1;u2];
ua=temp(1);
ub=temp(2);
uc=temp(3);

== matlab function saved3/电压控制离散化/controller1/MATLAB Function ==
  data: wloop input; Vdirect input; Switch input; t input; out output
function out = fcn(wloop,Vdirect,Switch,t)
step1time=0.1;
step2time=0.2;
Ustart=1;
direction=1;
if t<step1time
    y=0;
else
    switch Switch
        case 0
            if t<step2time
                y=Ustart*direction;
            else
                y=wloop;
            end
        case 1
            y=Vdirect;
        otherwise
            y=0;
    end
end
out=y;

== matlab function saved3/电压控制离散化/controller1/MATLAB Function1 ==
  data: u input; y output; t input
function y = fcn(u,t)
startTime=0.2;
if t>startTime
    y=u;
else
    y=0;
end

== matlab function saved3/电压控制离散化/controller1/MATLAB Function2 ==
  data: gate input; u input; y output
function y = fcn(gate,u)
if gate<100
    y=u;
else
    y=0;
end

== matlab function saved3/电压控制离散化/controller1/clack & park1 ==
  data: ua input; u1 output; ub input; uc input; t input; u2 output
function [u1,u2] = fcn(ua,ub,uc,t)
clack=2/3*[1 -1/2 -1/2;0 sqrt(3)/2 -sqrt(3)/2];
park=[cos(t) sin(t);-sin(t) cos(t)];
temp=park*clack*[ua;ub;uc];
u1=temp(1);
u2=temp(2);

== matlab function saved3/电压控制离散化/current seperator1/电流采样/A//D转换 10KHz2 ==
  data: u input; y output
function y = fcn(u)
bina=16; %二进制位数
deci=3; %小数位数
Max=2^bina;
uper=Max/10^deci/2;
out=fix(u*10^deci+0.5)/10^deci;
y = min(uper,abs(out))*sign(out);

== matlab function saved3/电压控制离散化/current seperator1/电流采样/A//D转换 10KHz3 ==
  data: u input; y output
function y = fcn(u)
bina=16; %二进制位数
deci=3; %小数位数
Max=2^bina;
uper=Max/10^deci/2;
out=fix(u*10^deci+0.5)/10^deci;
y = min(uper,abs(out))*sign(out);

== matlab function saved3/电压控制离散化/current seperator1/电流采样/A//D转换 10KHz4 ==
  data: u input; y output
function y = fcn(u)
bina=16; %二进制位数
deci=3; %小数位数
Max=2^bina;
uper=Max/10^deci/2;
out=fix(u*10^deci+0.5)/10^deci;
y = min(uper,abs(out))*sign(out);

== matlab function saved3/电压控制离散化/current seperator1/电流采样1/A//D转换 10KHz2 ==
  data: u input; y output
function y = fcn(u)
bina=16; %二进制位数
deci=2; %小数位数
Max=2^bina;
uper=Max/10^deci/2;
out=fix(u*10^deci+0.5)/10^deci;
y = min(uper,abs(out))*sign(out);

== matlab function saved3/电压控制离散化/current seperator1/电流采样1/A//D转换 10KHz3 ==
  data: u input; y output
function y = fcn(u)
bina=16; %二进制位数
deci=2; %小数位数
Max=2^bina;
uper=Max/10^deci/2;
out=fix(u*10^deci+0.5)/10^deci;
y = min(uper,abs(out))*sign(out);

== matlab function saved3/电压控制离散化/current seperator1/电流采样1/A//D转换 10KHz4 ==
  data: u input; y output
function y = fcn(u)
bina=16; %二进制位数
deci=2; %小数位数
Max=2^bina;
uper=Max/10^deci/2;
out=fix(u*10^deci+0.5)/10^deci;
y = min(uper,abs(out))*sign(out);

== matlab function saved3/电压控制离散化/inject estimater(digital)1/clack & park2 ==
  data: ua input; u1 output; ub input; uc input; t input; u2 output
function [u1,u2] = fcn(ua,ub,uc,t)
clack=2/3*[1 -1/2 -1/2;0 sqrt(3)/2 -sqrt(3)/2];
park=[cos(t) sin(t);-sin(t) cos(t)];
temp=park*clack*[ua;ub;uc];
u1=temp(1);
u2=temp(2);

== matlab function saved3/电压控制离散化/inject estimater(digital)1/鉴幅鉴相器(可选快速门滑窗)1 ==
  data: S1 input; A1 output; A2 output; S2 input; DP output; Fre input
function [A1,A2, DP] = fcn(S1,S2,Fre)
Ts=1e-4; %采样时间，其倒数需大于10倍探测信号频率
detPsi=Fre; %探测频率.需采样完整周期整数倍
LowPsi=Fre; %输入信号中的最低显著频率，若探测频率远大于该项，需前置高通滤波器
bufsize=2/LowPsi/Ts;
winSize=1; %滑窗步长
complexStyle=1+1j;
persistent buf1 buf2 round outBuf corebuf gate
if isempty(buf1)||isempty(round)
    buf1=zeros(1,bufsize);
    buf2=zeros(1,bufsize);
    corebuf=zeros(1,bufsize,'like',complexStyle);
    round=0;
    outBuf=[0,0,0];
    gate=0;
end
% 数据读取
if round>=bufsize
    round=0;
    gate=1;
end
buf1(round+1)=S1;
buf2(round+1)=S2;
% 数据处理
corebuf(round+1)=exp(-2*pi*1j*detPsi*round*Ts)*Ts;
if gate==1
    if mod(round+1,winSize)==0
        F1=0+0j;F2=0+0j;
        for n=0:bufsize-1
            F1=F1+buf1(n+1)*corebuf(n+1);
            F2=F2+buf2(n+1)*corebuf(n+1);
        end
        F1=F1*2/bufsize/Ts;F2=F2*2/bufsize/Ts;
        outBuf(1)=norm(F1);outBuf(2)=norm(F2);
        outBuf(3)=angle(F2/F1)*180/pi; %S2超前S1的相位
    end
end
% 更新与输出
round=round+1;
A1=outBuf(1);A2=outBuf(2);
DP=outBuf(3);

== matlab function saved3/电压控制离散化/inject estimater(digital)1/锁相器1 ==
  data: u input; the output; w output
function [the,w] = fcn(u)
% PI控制器部分
ts=1e-4;
kp=4; ki=350;
persistent intg
if isempty(intg)
    intg=0;
end
intg=intg+u*ts;
w = kp*u+ki*intg;

% 积分器部分
persistent intg2
if isempty(intg2)
    intg2=0;
end
intg2=intg2+w*ts;
the = intg2;

== matlab function saved3/电压控制离散化/inv(clack & park)2 ==
  data: u1 input; ua output; u2 input; t input; ub output; uc output
function [ua,ub,uc] = fcn(u1,u2,t)
invClack=3/2*[2/3 0;-1/3 sqrt(3)/3;-1/3 -sqrt(3)/3];
invPark=[cos(t) -sin(t);sin(t) cos(t)];
temp=invClack*invPark*[u1;u2];
ua=temp(1);
ub=temp(2);
uc=temp(3);

== matlab function saved3/电压控制离散化/w estimater1/clack1 ==
  data: ia input; iap output; ib input; ic input; ibe output
function [iap,ibe] = fcn(ia,ib,ic)
clack=2/3*[1 -1/2 -1/2;0 sqrt(3)/2 -sqrt(3)/2];
temp=clack*[ia;ib;ic];
iap=temp(1);
ibe=temp(2);

== matlab function saved3/电压控制离散化/w estimater1/invpark ==
  data: u1 input; ua output; u2 input; ub output; t input
function [ua,ub] = fcn(u1,u2,t)
invPark=[cos(t) -sin(t);sin(t) cos(t)];
temp=invPark*[u1;u2];
ua=temp(1);
ub=temp(2);

== matlab function saved3/电压控制离散化/w estimater1/磁链观测器 ==
  data: u input; y output
function y = fcn(u)
ts=1e-4;
R=0.1;
L=1.2e-3;
Psi_mm=0.1;
uob=[u(1);u(2)];
iob=[u(3);u(4)];

persistent x_1
if isempty(x_1)
    x_1=[0;0];
end
gamma=20000;
ita=x_1-L*iob;
err=Psi_mm^2-norm(ita)^2;
x=x_1 + (uob-iob*R+gamma*ita*err)*ts;
x_1=x;
v=(x-L*iob);
y = atan2(v(2),v(1))-0.0;
